simulink model "invertpen"  (R2022b)
settings: Solver=VariableStepAuto  StartTime=0.0  StopTime=10.0  RelTol=1e-3
values from neighbouring files (symbols this model uses):
  A = [0 1 0 0; 0 0 m*g/M 0; 0 0 0 1; 0 0 (M+m)*g/(M*l) 0]    [invertpen_script.m]    (also in optimal_a3.mat = [0 0 0 0 1 0 0 0 0 2.100456621 0 36.0401472471 ... (16 eleme; optimal_b2.mat = [0 0 0 0 1 0 0 0 0 2.100456621 0 36.0401472471 ... (16 eleme; optimal_b3.mat = [0 0 0 0 1 0 0 0 0 2.100456621 0 36.0401472471 ... (16 eleme; optimal_c2.mat = [0 0 0 0 1 0 0 0 0 2.100456621 0 36.0401472471 ... (16 eleme)
  B = [0;1/M;0;1/l/M]    [invertpen_script.m]    (also in optimal_a3.mat = [0 0.931879601156 0 2.82216717491]; optimal_b2.mat = [0 0.931879601156 0 2.82216717491]; optimal_b3.mat = [0 0.931879601156 0 2.82216717491]; optimal_c2.mat = [0 0.931879601156 0 2.82216717491])
  C = [1,0,0,0;0,0,1,0]    [invertpen_script.m]    (also in optimal_a3.mat = [1  0  0  0; 0  0  1  0]; optimal_b2.mat = [1  0  0  0; 0  0  1  0]; optimal_b3.mat = [1  0  0  0; 0  0  1  0]; optimal_c2.mat = [1  0  0  0; 0  0  1  0])
  g = 9.8    [invertpen_script.m]    (also in optimal_a3.mat; optimal_b2.mat; optimal_b3.mat; optimal_c2.mat)
  K = [0.4472,1.2429,-29.6951,-4.9864]    [invertpen_script.m]    (also in optimal_a3.mat = [5.47722557505 5.67413665606 -41.5732016325 -7.18210280699]; optimal_b2.mat = [0.316227766017 1.30734830298 -39.2540821539 -5.6989814793]; optimal_b3.mat = [0.316227766017 2.07846129293 -79.7094943701 -8.19724303463]; optimal_c2.mat = [10 15.4667752933 -129.988737607 -14.582347098])
  L = -1*FO_observer    [invertpen_script.m]    (also in optimal_a3.mat = [37.9755841509  0.0115288283108; 360.356054275  2.8721224085; optimal_b2.mat = [37.9755841509  0.0115288283108; 360.356054275  2.8721224085; optimal_b3.mat = [37.9755841509  0.0115288283108; 360.356054275  2.8721224085; optimal_c2.mat = [37.9755841509  0.0115288283108; 360.356054275  2.8721224085)
  l = 0.3302    [invertpen_script.m]    (also in optimal_a3.mat; optimal_b2.mat; optimal_b3.mat; optimal_c2.mat)
  m = 0.2300    (= 0.23)    [invertpen_script.m]    (also in optimal_a3.mat; optimal_b2.mat; optimal_b3.mat; optimal_c2.mat)
  M = 1.0731    [invertpen_script.m]    (also in optimal_a3.mat; optimal_b2.mat; optimal_b3.mat; optimal_c2.mat)
settings Model: Creator=kevin  LastModifiedBy=kevin
settings SolverCC: AlgebraicLoopSolver=TrustRegion
settings DebuggingCC: UnconnectedInputMsg=warning  UnconnectedOutputMsg=warning  UnconnectedLineMsg=warning  SFMachineParentedDataDiag=warning
settings ModelReferenceCC: EnableRefExpFcnMdlSchedulingChecks=on

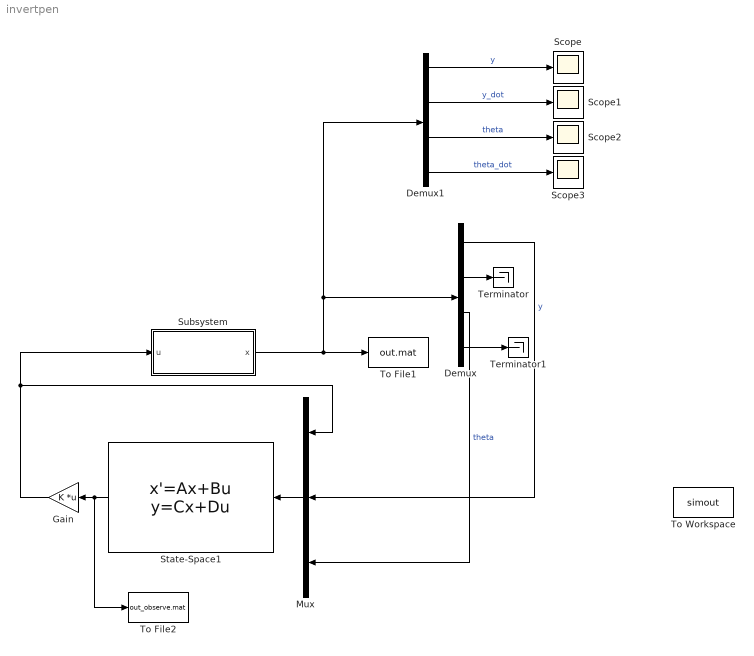
== system invertpen ==
  Demux : Demux
  Demux1 : Demux
  Gain : Gain  Gain=K  Multiplication=Matrix(K*u)
  Mux : Mux  Inputs=3
  Scope{,1..3} (4 alike) : Scope
  State-Space1 : StateSpace  A=A-L*C  B=[B L]  C=eye(4)  D=zeros(4,3)  InitialCondition=[0;0;0;0]
  Subsystem : Subsystem
  Terminator : Terminator
  Terminator1 : Terminator
  To File1 : ToFile  Filename=out.mat  MatrixName=output
  To File2 : ToFile  Filename=out_observe.mat  MatrixName=output_o
  To Workspace : ToWorkspace  VariableName=simout  SaveFormat=Timeseries  SampleTime=-1
  wires:
  Demux/3 -> Mux/3  "theta"
  Demux/1 -> Mux/2  "y"
  Demux1/4 -> Scope3/1  "theta_dot"
  Demux1/1 -> Scope/1  "y"
  Demux1/2 -> Scope1/1  "y_dot"
  Demux1/3 -> Scope2/1  "theta"
  Mux/1 -> State-Space1/1
  Gain/1 -> Subsystem/1(u), Mux/1
  Subsystem/1(x) -> To File1/1, Demux1/1, Demux/1
  State-Space1/1 -> To File2/1, Gain/1
  Demux/2 -> Terminator/1
  Demux/4 -> Terminator1/1

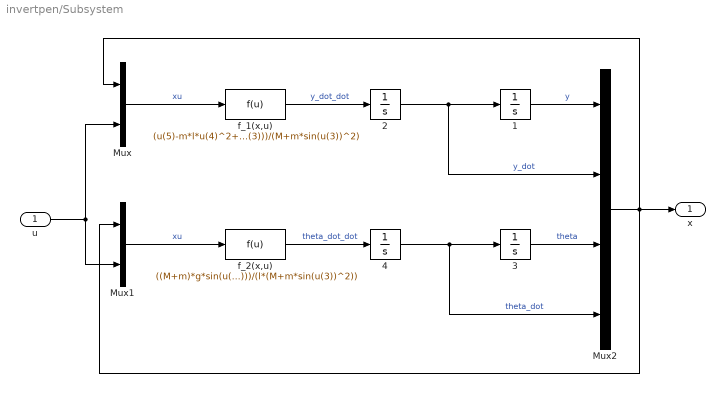
== system invertpen/Subsystem ==
  u : Inport
  1 : Integrator  InitialCondition=0.5
  2 : Integrator  InitialCondition=0.1
  3 : Integrator  InitialCondition=0.175
  4 : Integrator
  Mux : Mux  Inputs=2
  Mux1 : Mux  Inputs=2
  Mux2 : Mux
  f_1(x,u) : Fcn  Expr=(u(5)-m*l*u(4)^2+m*g*cos(u(3))*sin(u(3)))/(M+m*sin(u(3))^2)
  f_2(x,u) : Fcn  Expr=((M+m)*g*sin(u(3))+u(5)*cos(u(3))-m*l*u(4)^2*sin(u(3))*cos(u(3)))/(l*(M+m*sin(u(3))^2))
  x : Outport
  wires:
  u/1 -> Mux1/2, Mux/2
  Mux/1 -> f_1(x,u)/1  "xu"
  Mux1/1 -> f_2(x,u)/1  "xu"
  3/1 -> Mux2/3  "theta"
  1/1 -> Mux2/1  "y"
  f_2(x,u)/1 -> 4/1  "theta_dot_dot"
  4/1 -> Mux2/4, 3/1  "theta_dot"
  f_1(x,u)/1 -> 2/1  "y_dot_dot"
  2/1 -> Mux2/2, 1/1  "y_dot"
  Mux2/1 -> x/1, Mux/1, Mux1/1
